simulink model "Q3"  (R2020b)
settings: Solver=VariableStepAuto  StartTime=0.0  StopTime=30  RelTol=1e-3
undefined symbols (not defined in the file): A_num, B_num, C_num, k1_integ, k2_integ
settings Model: Creator=asus  LastModifiedBy=asus

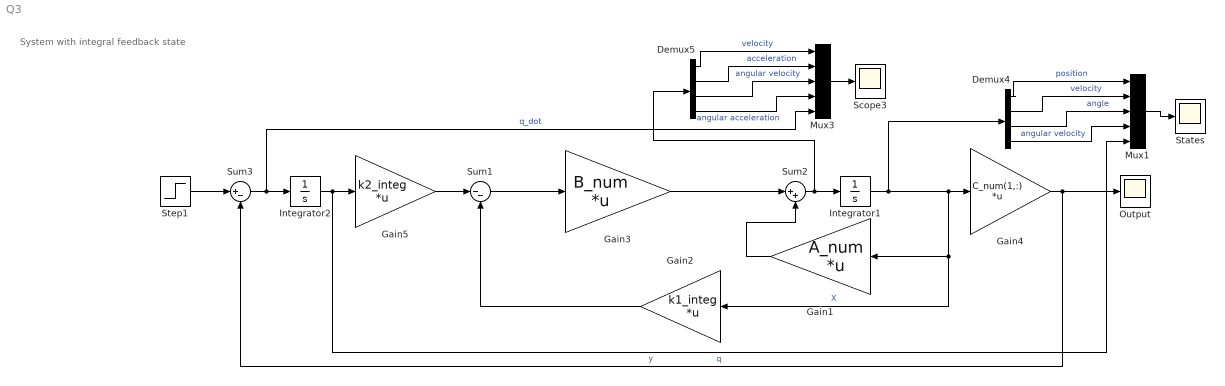
== system Q3 ==
  note: System with integral feedback state
  Demux4 : Demux
  Demux5 : Demux
  Gain1 : Gain  Gain=A_num  Multiplication=Matrix(K*u)
  Gain2 : Gain  Gain=k1_integ  Multiplication=Matrix(K*u)
  Gain3 : Gain  Gain=B_num  Multiplication=Matrix(K*u)
  Gain4 : Gain  Gain=C_num(1,:)  Multiplication=Matrix(K*u)
  Gain5 : Gain  Gain=k2_integ  Multiplication=Matrix(K*u)
  Integrator1 : Integrator
  Integrator2 : Integrator
  Mux1 : Mux  Inputs=5
  Mux3 : Mux  Inputs=5
  Output : Scope
  Scope3 : Scope
  States : Scope
  Step1 : Step  After=0.1  SampleTime=0
  Sum1 : Sum  Inputs=|--
  Sum2 : Sum  Inputs=|++
  Sum3 : Sum  Inputs=|+-
  wires:
  Demux5/3 -> Mux3/3  "angular velocity"
  Sum1/1 -> Gain3/1
  Step1/1 -> Sum3/1
  Demux5/2 -> Mux3/2  "acceleration"
  Demux4/3 -> Mux1/3  "angle"
  Gain3/1 -> Sum2/1
  Demux4/1 -> Mux1/1  "position"
  Demux4/2 -> Mux1/2  "velocity"
  Integrator1/1 -> Gain2/1, Gain1/1, Gain4/1, Demux4/1  "X"
  Integrator2/1 -> Mux1/5, Gain5/1  "q"
  Demux4/4 -> Mux1/4  "angular velocity"
  Demux5/4 -> Mux3/4  "angular acceleration"
  Mux1/1 -> States/1
  Demux5/1 -> Mux3/1  "velocity"
  Sum2/1 -> Demux5/1, Integrator1/1
  Sum3/1 -> Mux3/5, Integrator2/1  "q_dot"
  Gain4/1 -> Sum3/2, Output/1  "y"
  Gain2/1 -> Sum1/2
  Gain1/1 -> Sum2/2
  Gain5/1 -> Sum1/1
  Mux3/1 -> Scope3/1
